simulink model "simulation"  (R2017a)
settings: Solver=ode1  StartTime=0.0  StopTime=50.0  RelTol=1e-3
settings Model: Creator=arthur  LastModifiedBy=arthur

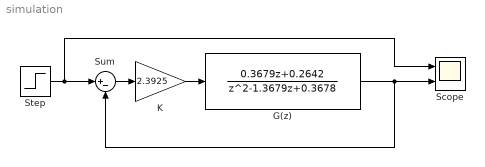
== system simulation ==
  G(z) : DiscreteTransferFcn  Numerator=[0.3679 0.2642]  Denominator=[1 -1.3679 0.3678]
  K : Gain  Gain=2.3925
  Scope : Scope  NumInputPorts=2
  Step : Step  SampleTime=1
  Sum : Sum  Inputs=|+-
  wires:
  K/1 -> G(z)/1
  Sum/1 -> K/1
  Step/1 -> Scope/1, Sum/1
  G(z)/1 -> Sum/2, Scope/2
